simulink model "Controls_Finalproject_1f_linear_with_integrator"  (R2015a)
settings: Solver=ode45  StartTime=0.0  StopTime=1000.0  RelTol=1e-3
values from neighbouring files (symbols this model uses):
  A = [ 0 1 0 0 0 0 0; 0 0 -(m1*g)/M 0 -m2*g/M 0 0; 0 0 0 1 0 0 0; 0 0 -(M+m1)*g/(M*l1) 0 -m2*g/(M*l1) 0 0; 0 0 0 0 0 1 0; 0 0 -m1*g/(M*l2) 0 -(M+m2)*g/(M*l2) 0 0; -1 0 0 0 0 0 0]    [linear_observer_testpiece.m]    (also in nonlinear_observer_testpiece.m)
  AKL = AKL4    [linear_observer_testpiece.m]    (also in nonlinear_observer_testpiece.m = AKL1)
  B = [0; 1/M; 0; 1/(M*l1); 0; 1/(M*l2); 0]    [linear_observer_testpiece.m]    (also in nonlinear_observer_testpiece.m)
  BL = BL4    [linear_observer_testpiece.m]    (also in nonlinear_observer_testpiece.m = BL1)
  C = C4    [linear_observer_testpiece.m]    (also in nonlinear_observer_testpiece.m = C1)
  CO = eye(6)    [linear_observer_testpiece.m]    (also in nonlinear_observer_testpiece.m)
  D = D4    [linear_observer_testpiece.m]    (also in nonlinear_observer_testpiece.m = D1)
  DO = DO4    [linear_observer_testpiece.m]    (also in nonlinear_observer_testpiece.m = DO1)
  X0 = X04    [linear_observer_testpiece.m]    (also in nonlinear_observer_testpiece.m = X01)
undefined symbols (not defined in the file or in its folder): K
settings Model: Creator=Aditya Earanky  LastModifiedBy=Aditya Earanky

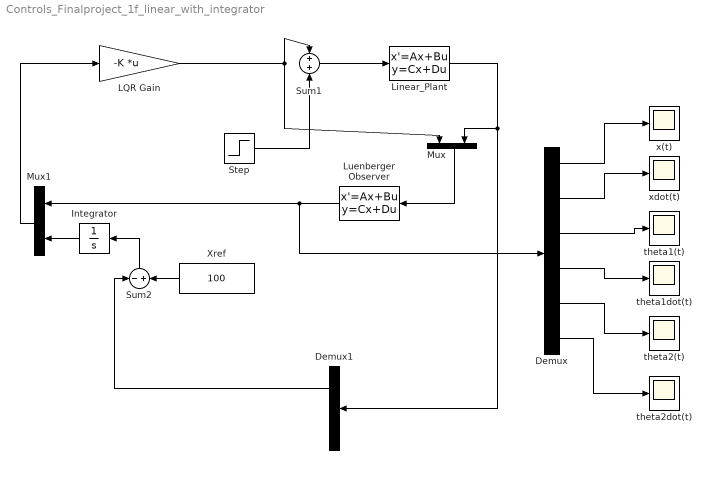
== system Controls_Finalproject_1f_linear_with_integrator ==
  Demux : Demux  Outputs=6
  Demux1 : Demux  Outputs=2
  Integrator : Integrator
  LQR Gain : Gain  Gain=-K  Multiplication=Matrix(K*u) (u vector)
  Linear_Plant : StateSpace  A=A  B=B  C=C  D=D  X0=X0
  Luenberger Observer : StateSpace  A=AKL  B=BL  C=CO  D=DO  X0=0
  Mux : Mux  Inputs=2
  Mux1 : Mux  Inputs=2
  Step : Step  SampleTime=0
  Sum1 : Sum
  Sum2 : Sum  Inputs=-+
  Xref : Constant  Value=100
  theta1(t) : Scope
      settings: TimeRange=1000  YMin=0  YMax=0.07  SaveName=ScopeData3
  theta1dot(t) : Scope
      settings: TimeRange=1000  YMin=0  YMax=0.07  SaveName=ScopeData5
  theta2(t) : Scope
      settings: TimeRange=1000  YMin=0  YMax=0.07  SaveName=ScopeData6
  theta2dot(t) : Scope
      settings: TimeRange=1000  YMin=0  YMax=0.07  SaveName=ScopeData7
  x(t) : Scope
      settings: TimeRange=1000  YMin=-1  YMax=1  SaveName=ScopeData2
  xdot(t) : Scope
      settings: TimeRange=1000  YMin=0  YMax=0.07  SaveName=ScopeData4
  wires:
  Linear_Plant/1 -> Demux1/1, Mux/2
  Mux/1 -> Luenberger Observer/1
  Demux/1 -> x(t)/1
  Sum2/1 -> Integrator/1
  Luenberger Observer/1 -> Demux/1, Mux1/1
  Integrator/1 -> Mux1/2
  Mux1/1 -> LQR Gain/1
  LQR Gain/1 -> Mux/1, Sum1/1
  Xref/1 -> Sum2/2
  Demux/2 -> xdot(t)/1
  Demux/3 -> theta1(t)/1
  Demux/4 -> theta1dot(t)/1
  Demux/5 -> theta2(t)/1
  Demux/6 -> theta2dot(t)/1
  Step/1 -> Sum1/2
  Sum1/1 -> Linear_Plant/1
  Demux1/1 -> Sum2/1
